simulink model "mod1"  (R2016b)
settings: Solver=VariableStepAuto  StartTime=0.0  StopTime=1.2  RelTol=1e-3
values from neighbouring files (symbols this model uses):
  f = 120    [Cons.m]
  Kconv = 7.576    [Cons.m]
  Ki = 43.2/1000    (= 0.0432)    [Cons.m]
  Kred = 35.9    [Cons.m]
  meq = 120    [Cons.m]
  rpignon = 21*0.8/(2*1000)    (= 0.0084)    [Cons.m]
settings Model: Creator=antoine.martin  LastModifiedBy=canar

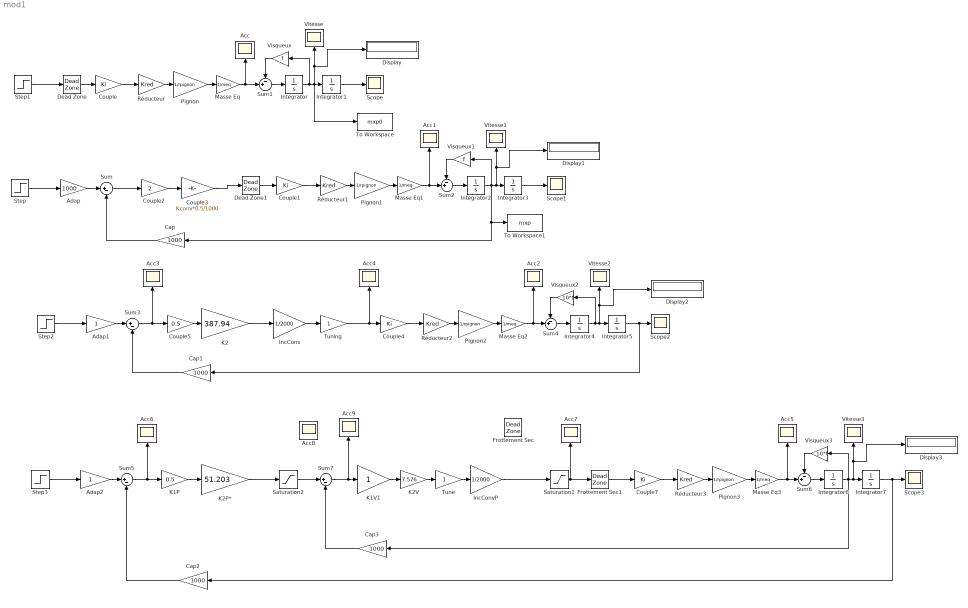
== system mod1 ==
  Acc{,1..9} (10 alike) : Scope
  Adap : Gain  Gain=1000
  Adap1 : Gain
  Adap2 : Gain
  Cap{,1..3} (4 alike) : Gain  Gain=1000
  Couple{,1,4,7} (4 alike) : Gain  Gain=Ki
  Couple2 : Gain  Gain=2
  Couple3 : Gain  Gain=Kconv*0.5/1000
  Couple5 : Gain  Gain=0.5
  Dead Zone : DeadZone  LowerValue=-0.05  UpperValue=0.05  SaturateOnIntegerOverflow=on
  Dead Zone1 : DeadZone  LowerValue=-0.05  UpperValue=0.05  SaturateOnIntegerOverflow=on
  Display{,1..3} (4 alike) : Display
  Frottement Sec : DeadZone  LowerValue=-0.0021  UpperValue=0.0021  SaturateOnIntegerOverflow=on
  Frottement Sec1 : DeadZone  LowerValue=-0.01  UpperValue=0.01  SaturateOnIntegerOverflow=on
  IncConv : Gain  Gain=1/2000
  IncConvP : Gain  Gain=1/2000
  Integrator{,1..7} (8 alike) : Integrator
  K1P : Gain  Gain=0.5
  K1V1 : Gain
  K2 : Gain  Gain=387.94
  K2P* : Gain  Gain=51.203
  K2V : Gain  Gain=7.576
  Masse Eq{,1..3} (4 alike) : Gain  Gain=1/meq
  Pignon{,1..3} (4 alike) : Gain  Gain=1/rpignon
  Réducteur{,1..3} (4 alike) : Gain  Gain=Kred
  Saturation1 : Saturate
  Saturation2 : Saturate  UpperLimit=135  LowerLimit=-135
  Scope{,1..3} (4 alike) : Scope
  Step : Step  Time=0.1  After=0.1  SampleTime=0
  Step1 : Step  Time=0.1  After=0.2  SampleTime=0
  Step2 : Step  Time=0.1  After=4  SampleTime=0
  Step3 : Step  Time=0.1  After=25  SampleTime=0
  Sum{,3,5,7} (4 alike) : Sum  Inputs=|+-
  Sum{1..2,4,6} (4 alike) : Sum  Inputs=-+|
  To Workspace : ToWorkspace  VariableName=mxp0  SaveFormat=Timeseries  SampleTime=-1
  To Workspace1 : ToWorkspace  VariableName=mxp  SaveFormat=Timeseries  SampleTime=-1
  Tune : Gain
  Tuning : Gain
  Visqueux : Gain  Gain=f
  Visqueux1 : Gain  Gain=f
  Visqueux2 : Gain  Gain=10*f
  Visqueux3 : Gain  Gain=10*f
  Vitesse{,1..3} (4 alike) : Scope
  wires:
  Step/1 -> Adap/1
  Adap/1 -> Sum/1
  Cap/1 -> Sum/2
  Pignon/1 -> Masse Eq/1
  Integrator/1 -> Visqueux/1, To Workspace/1, Display/1, Vitesse/1, Integrator1/1
  Integrator1/1 -> Scope/1
  Sum1/1 -> Integrator/1
  Visqueux/1 -> Sum1/1
  Masse Eq/1 -> Sum1/2, Acc/1
  Réducteur/1 -> Pignon/1
  Step1/1 -> Dead Zone/1
  Couple/1 -> Réducteur/1
  Pignon1/1 -> Masse Eq1/1
  Integrator2/1 -> To Workspace1/1, Cap/1, Visqueux1/1, Display1/1, Vitesse1/1, Integrator3/1
  Integrator3/1 -> Scope1/1
  Sum2/1 -> Integrator2/1
  Visqueux1/1 -> Sum2/1
  Masse Eq1/1 -> Sum2/2, Acc1/1
  Réducteur1/1 -> Pignon1/1
  Couple1/1 -> Réducteur1/1
  Sum/1 -> Couple2/1
  Couple2/1 -> Couple3/1
  Step2/1 -> Adap1/1
  Adap1/1 -> Sum3/1
  Cap1/1 -> Sum3/2
  Pignon2/1 -> Masse Eq2/1
  Integrator4/1 -> Visqueux2/1, Display2/1, Vitesse2/1, Integrator5/1
  Integrator5/1 -> Cap1/1, Scope2/1
  Sum4/1 -> Integrator4/1
  Visqueux2/1 -> Sum4/1
  Masse Eq2/1 -> Sum4/2, Acc2/1
  Réducteur2/1 -> Pignon2/1
  Couple4/1 -> Réducteur2/1
  Sum3/1 -> Acc3/1, Couple5/1
  K2/1 -> IncConv/1
  Couple5/1 -> K2/1
  IncConv/1 -> Tuning/1
  Tuning/1 -> Acc4/1, Couple4/1
  Step3/1 -> Adap2/1
  Adap2/1 -> Sum5/1
  Cap2/1 -> Sum5/2
  Pignon3/1 -> Masse Eq3/1
  Integrator6/1 -> Cap3/1, Visqueux3/1, Display3/1, Vitesse3/1, Integrator7/1
  Integrator7/1 -> Cap2/1, Scope3/1
  Sum6/1 -> Integrator6/1
  Visqueux3/1 -> Sum6/1
  Masse Eq3/1 -> Sum6/2, Acc5/1
  Réducteur3/1 -> Pignon3/1
  Couple7/1 -> Réducteur3/1
  Sum5/1 -> Acc6/1, K1P/1
  K1P/1 -> K2P*/1
  K1V1/1 -> K2V/1
  K2V/1 -> Tune/1
  Cap3/1 -> Sum7/2
  Tune/1 -> IncConvP/1
  IncConvP/1 -> Saturation1/1
  Saturation1/1 -> Frottement Sec1/1, Acc7/1
  K2P*/1 -> Saturation2/1
  Sum7/1 -> Acc9/1, K1V1/1
  Saturation2/1 -> Sum7/1
  Frottement Sec1/1 -> Couple7/1
  Dead Zone/1 -> Couple/1
  Dead Zone1/1 -> Couple1/1
  Couple3/1 -> Dead Zone1/1
